simulink model "fivephase_inverter_without_speed_control_v66"  (R2019b)
settings: Solver=FixedStepAuto  StartTime=0.0  StopTime=0.2  FixedStep=t_s  MaxStep=1e-4  RelTol=1e-3
values from neighbouring files (symbols this model uses):
  pulse = zeros(5,7,10)    [run_simulink_model.m]
  T_load_time = 0    [run_simulink_model.m]
  t_s = 1e-6    (= 1e-06)    [run_simulink_model.m]
  w_init = 70*pi    (= 219.911485751)    [run_simulink_model.m]
  w_rev_time = 3    [run_simulink_model.m]
  w_set = 70*pi    (= 219.911485751)    [run_simulink_model.m]
libraries: powerlib x49, simulink x6, powerlib_meascontrol x5, simulink_extras x1
settings Model: Creator=user  LastModifiedBy=user
settings SolverCC: AlgebraicLoopSolver=LineSearch
settings DataIOCC: ReturnWorkspaceOutputs=off
settings DebuggingCC: ArithmeticOperatorsInVariantConditions=warning
settings SFSimCC: SimUseLocalCustomCode=off  CustomCodeUndefinedFunction=UseInterfaceOnly
settings RTWCC: RTWUseLocalCustomCode=off

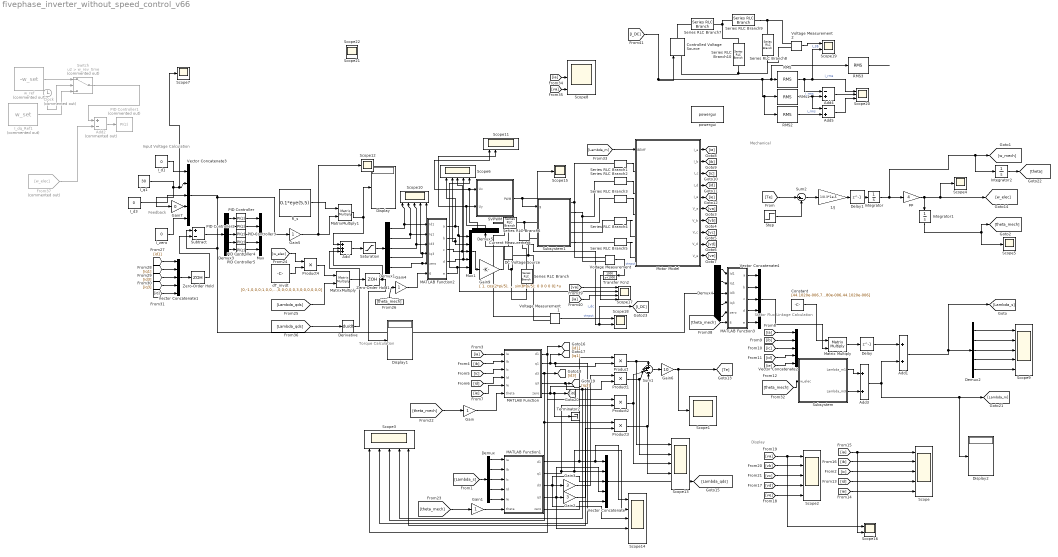
== system fivephase_inverter_without_speed_control_v66 ==
  note: Input Voltage Calculation
  note: Feedback
  note: Torque Calculation
  note: Stator Flux Linkage Calculation
  note: Mechanical
  note: Display
  1/J : Gain  Gain=1/0.3*1e-5
  Add : Sum  Inputs=+++
  Add1 : Sum
  Add2 : Sum  Commented=on  Inputs=+-
  Add3 : Sum
  Add4 : Sum  Inputs=-+
  Add5 : Sum  Inputs=-+
  Clock : Clock  Commented=on
  Constant : Constant  Value=[44.1020e-006,7.6280e-006,-24.9980e-006,-24.9980e-006,7.6280e-006;7.6280e-006,44.1020e-006,7.6280e-006,-24.9980e-006,-24.9980e-006;-24.9980e-006,7.6280e-006, 44.1020e-006,7.6280e-006,-24.9980e-006;-24.9980e-006,-24.9980e-006,7.6280e-006,44.1020e-006,7.6280e-006;7.6280e-006 ,-24.9980e-006,-24.9980e-006,7.6280e-006,44.1020e-006]  SampleTime=-1
  Controlled Voltage Source : powerlib/Electrical Sources/Controlled Voltage Source  Initialize=on  Source_Type=AC  Amplitude=0  Phase=0  Frequency=0  Measurements=None
      settings: SourceProductName=Simscape Electrical
  Current Measurement : powerlib/Measurements/Current Measurement  PhasorSimulation=off  OutputType=Complex  PSBequivalent=0
      settings: SourceProductName=Simscape Electrical
  DC Voltage Source : powerlib/Electrical Sources/DC Voltage Source  Amplitude=80  Measurements=None
      settings: SourceProductName=Simscape Electrical
  Delay : Delay  DelayLength=1  InitialCondition=1
  Delay1 : Delay  DelayLength=1  InitialCondition=35/2*pi
  Demux{,1..4} (5 alike) : Demux  Outputs=5
  Demux5 : Demux  Outputs=3
  Derivative : Derivative  CoefficientInTFapproximation=1e-5
  Display : Display
  Display1 : Display
  Display2 : Display
  From37 : From  Commented=on  GotoTag=w_elec
  Gain{,1,4..5} (4 alike) : Gain
  Gain2 : Gain  Gain=3
  Gain3 : Gain  Gain=3
  Gain6 : Gain  Gain=10
  Gain7 : Gain  Gain=0
  Gain9 : Gain  Gain=[ 1, cos(2*pi/5), cos(4*pi/5), cos(6*pi/5), cos(8*pi/5); 0, sin(2*pi/5),sin(4*pi/5), sin(6*pi/5), sin(8*pi/5); 0 0 0 0 0]  Multiplication=Matrix(K*u) (u vector)  SaturateOnIntegerOverflow=on  OutDataTypeStr=Inherit: Same as input  ParamDataTypeStr=Inherit: Same as input
  I_d1 : Constant  Value=0
  I_d3 : Constant  Value=0
  I_dq_Ref1 : Constant  Commented=on  Value=w_set
  I_q1 : Constant  Value=30
  I_zero : Constant  Value=0
  Integrator : Integrator  InitialCondition=w_init/4
  Integrator1 : Integrator
  Integrator2 : Integrator
  MATLAB Function : MATLAB Function  TreatAsAtomicUnit=on
  MATLAB Function1 : MATLAB Function  TreatAsAtomicUnit=on
  MATLAB Function2 : MATLAB Function  TreatAsAtomicUnit=on
  MATLAB Function3 : MATLAB Function  TreatAsAtomicUnit=on
  Matrix Multiply : Product  Multiplication=Matrix(*)
  MatrixMultiply : Product  Multiplication=Matrix(*)
  MatrixMultiply1 : Product  Multiplication=Matrix(*)
  Motor Model : Subsystem
  Mux : Mux  Inputs=5
  Mux1 : Mux  Inputs=5
  PID Controller{,2..5} (5 alike) : simulink/Continuous/PID Controller  Controller=PI  Form=Parallel  TimeDomain=Discrete-time  SampleTime=t_s  IntegratorMethod=Forward Euler  FilterMethod=Forward Euler  ControllerParametersSource=internal  P=5  I=5  D=0  UseFilter=on  N=100  TunerSelectOption=Transfer Function Based (PID Tuner App)  InitialConditionSource=internal  InitialConditionForIntegrator=0  InitialConditionForFilter=0  DifferentiatorICPrevScaledInput=0  ExternalReset=none  TrackingMode=off  Kt=1  LimitOutput=off  UpperSaturationLimit=75  LowerSaturationLimit=-75  LinearizeAsGain=on  AntiWindupMode=clamping  Kb=1  POutMin=[]  POutMax=[]  IOutMin=[]  IOutMax=[]  DOutMin=[]  DOutMax=[]  NOutMin=[]  NOutMax=[]  SumOutMin=[]  SumOutMax=[]  SaturationOutMin=[]  SaturationOutMax=[]  PParamMin=[]  PParamMax=[]  IParamMin=[]  IParamMax=[]  DParamMin=[]  DParamMax=[]  NParamMin=[]  NParamMax=[]  KbParamMin=[]  KbParamMax=[]  KtParamMin=[]  KtParamMax=[]  KbOutMin=[]  KbOutMax=[]  KtOutMin=[]  KtOutMax=[]  IntegratorOutMin=[]  IntegratorOutMax=[]  FilterOutMin=[]  FilterOutMax=[]  SumI1OutMin=[]  SumI1OutMax=[]  SumI2OutMin=[]  SumI2OutMax=[]  SumI3OutMin=[]  SumI3OutMax=[]  SumI4OutMin=[]  SumI4OutMax=[]  SumDOutMin=[]  SumDOutMax=[]  DifferentiatorOutMin=[]  DifferentiatorOutMax=[]  FilterDiffOutCoefMin=[]  FilterDiffOutCoefMax=[]  ReciprocalOutMin=[]  ReciprocalOutMax=[]  SumDenOutMin=[]  SumDenOutMax=[]  SumNumOutMin=[]  SumNumOutMax=[]  DivideOutMin=[]  DivideOutMax=[]  IntegratorContinuousStateAttributes=''  IntegratorStateMustResolveToSignalObject=off  IntegratorRTWStateStorageClass=Auto  FilterContinuousStateAttributes=''  FilterStateMustResolveToSignalObject=off  FilterRTWStateStorageClass=Auto  ParallelPVariant=InternalParameters  IdealPVariant=Disabled  IVariant=InternalParameters  DVariant=Disabled  IntegratorVariant=Discrete  SatVariant=Disabled  AWVariant=Passthrough  PCopyVariant=Disabled  TRVariant=Disabled  FdbkBlocksVariant=Forward  IdealPFdbkVariant=Disabled  SatFdbkVariant=Disabled  DerivativeFilterVariant=Disabled  NVariant=Disabled  NCopyVariant=Disabled_SignalSpec  FilterICVariant=Disabled  IntegratorICVariant=InternalICs  ExternalResetVariant=Disabled  TRSumVariant=Passthrough  SumFdbkVariant=Disabled  SumVariant=Sum_PI
  PID Controller1 : simulink/Continuous/PID Controller  Commented=on  Controller=PI  Form=Parallel  TimeDomain=Discrete-time  SampleTime=t_s  IntegratorMethod=Forward Euler  FilterMethod=Forward Euler  ControllerParametersSource=internal  P=2  I=30  D=0  UseFilter=on  N=100  TunerSelectOption=Transfer Function Based (PID Tuner App)  InitialConditionSource=internal  InitialConditionForIntegrator=0  InitialConditionForFilter=0  DifferentiatorICPrevScaledInput=0  ExternalReset=none  TrackingMode=off  Kt=1  LimitOutput=on  UpperSaturationLimit=80  LowerSaturationLimit=-80  LinearizeAsGain=on  AntiWindupMode=clamping  Kb=1  POutMin=[]  POutMax=[]  IOutMin=[]  IOutMax=[]  DOutMin=[]  DOutMax=[]  NOutMin=[]  NOutMax=[]  SumOutMin=[]  SumOutMax=[]  SaturationOutMin=[]  SaturationOutMax=[]  PParamMin=[]  PParamMax=[]  IParamMin=[]  IParamMax=[]  DParamMin=[]  DParamMax=[]  NParamMin=[]  NParamMax=[]  KbParamMin=[]  KbParamMax=[]  KtParamMin=[]  KtParamMax=[]  KbOutMin=[]  KbOutMax=[]  KtOutMin=[]  KtOutMax=[]  IntegratorOutMin=[]  IntegratorOutMax=[]  FilterOutMin=[]  FilterOutMax=[]  SumI1OutMin=[]  SumI1OutMax=[]  SumI2OutMin=[]  SumI2OutMax=[]  SumI3OutMin=[]  SumI3OutMax=[]  SumI4OutMin=[]  SumI4OutMax=[]  SumDOutMin=[]  SumDOutMax=[]  DifferentiatorOutMin=[]  DifferentiatorOutMax=[]  FilterDiffOutCoefMin=[]  FilterDiffOutCoefMax=[]  ReciprocalOutMin=[]  ReciprocalOutMax=[]  SumDenOutMin=[]  SumDenOutMax=[]  SumNumOutMin=[]  SumNumOutMax=[]  DivideOutMin=[]  DivideOutMax=[]  IntegratorContinuousStateAttributes=''  IntegratorStateMustResolveToSignalObject=off  IntegratorRTWStateStorageClass=Auto  FilterContinuousStateAttributes=''  FilterStateMustResolveToSignalObject=off  FilterRTWStateStorageClass=Auto  ParallelPVariant=InternalParameters  IdealPVariant=Disabled  IVariant=InternalParameters  DVariant=Disabled  IntegratorVariant=Discrete  SatVariant=Enabled  AWVariant=DiscClampingParallel  PCopyVariant=Disabled  TRVariant=Disabled  FdbkBlocksVariant=Forward  IdealPFdbkVariant=Disabled  SatFdbkVariant=Disabled  DerivativeFilterVariant=Disabled  NVariant=Disabled  NCopyVariant=Disabled_SignalSpec  FilterICVariant=Disabled  IntegratorICVariant=InternalICs  ExternalResetVariant=Disabled  TRSumVariant=Passthrough  SumFdbkVariant=Disabled  SumVariant=Sum_PI
  Product{,1..4} (5 alike) : Product
  RMS : powerlib_meascontrol/Measurements/RMS  TrueRMS=off  Freq=350  RMSInit=0  Ts=0
      settings: SourceProductName=Simscape Electrical
  RMS1 : powerlib_meascontrol/Measurements/RMS  TrueRMS=off  Freq=700  RMSInit=0  Ts=0
      settings: SourceProductName=Simscape Electrical
  RMS2 : powerlib_meascontrol/Measurements/RMS  TrueRMS=off  Freq=15000  RMSInit=0  Ts=0
      settings: SourceProductName=Simscape Electrical
  RMS3 : powerlib_meascontrol/Measurements/RMS  TrueRMS=off  Freq=7  RMSInit=0  Ts=0
      settings: SourceProductName=Simscape Electrical
  R_s : Constant  Value=0.1*eye(5,5)
  SVPWM : Subsystem  mask{Fc=15000, Vdc=80, Ts=t_s}
      mask prompts: Fc "PWM frequency"; Vdc "DC bus voltage"; Ts "Sampling time"
  Saturation : Saturate  UpperLimit=50  LowerLimit=-50
  Scope{,2..3,6,9..11,13..14} (9 alike) : Scope  NumInputPorts=5
  Scope{1,4..5,7,12,15,21..22} (8 alike) : Scope
  Scope16 : Scope  NumInputPorts=2
  Scope17 : Scope  NumInputPorts=4
  Scope18 : Scope  NumInputPorts=2
  Scope19 : Scope  NumInputPorts=2
  Scope20 : Scope  NumInputPorts=3
  Scope8 : Scope  NumInputPorts=3
  Series RLC Branch : powerlib/Elements/Series RLC Branch  LConnTagsString=__new0  RConnTagsString=__new0  BranchType=RC  Resistance=1e-12  Inductance=1e-3  SetiL0=off  InitialCurrent=0  Capacitance=100e-6  Setx0=off  InitialVoltage=0  Measurements=None
      settings: SourceProductName=Simscape Electrical
  Series RLC Branch{1..5} (5 alike) : powerlib/Elements/Series RLC Branch  LConnTagsString=__new0  RConnTagsString=__new0  BranchType=R  Resistance=1e-2  Inductance=1e-3  SetiL0=off  InitialCurrent=0  Capacitance=1e-6  Setx0=off  InitialVoltage=0  Measurements=None
      settings: SourceProductName=Simscape Electrical
  Series RLC Branch10 : powerlib/Elements/Series RLC Branch  LConnTagsString=__new0  RConnTagsString=__new0  BranchType=C  Resistance=50  Inductance=125.6e-3  SetiL0=off  InitialCurrent=0  Capacitance=5.025e-6  Setx0=off  InitialVoltage=0  Measurements=None
      settings: SourceProductName=Simscape Electrical
  Series RLC Branch6 : powerlib/Elements/Series RLC Branch  LConnTagsString=__new0  RConnTagsString=__new0  BranchType=L  Resistance=1e-12  Inductance=1e-3  SetiL0=off  InitialCurrent=0  Capacitance=100e-6  Setx0=off  InitialVoltage=0  Measurements=None
      settings: SourceProductName=Simscape Electrical
  Series RLC Branch7 : powerlib/Elements/Series RLC Branch  LConnTagsString=__new0  RConnTagsString=__new0  BranchType=R  Resistance=50  Inductance=1e-3  SetiL0=off  InitialCurrent=0  Capacitance=1e-6  Setx0=off  InitialVoltage=0  Measurements=None
      settings: SourceProductName=Simscape Electrical
  Series RLC Branch8 : powerlib/Elements/Series RLC Branch  LConnTagsString=__new0  RConnTagsString=__new0  BranchType=R  Resistance=50  Inductance=1e-3  SetiL0=off  InitialCurrent=0  Capacitance=1e-6  Setx0=off  InitialVoltage=0  Measurements=None
      settings: SourceProductName=Simscape Electrical
  Series RLC Branch9 : powerlib/Elements/Series RLC Branch  LConnTagsString=__new0  RConnTagsString=__new0  BranchType=L  Resistance=50  Inductance=12.56e-3  SetiL0=off  InitialCurrent=0  Capacitance=1e-6  Setx0=off  InitialVoltage=0  Measurements=None
      settings: SourceProductName=Simscape Electrical
  Step : Step  Time=T_load_time  After=26.07  SampleTime=0
  Subsystem : Subsystem
  Subsystem1 : Subsystem
  Subtract : Sum  Inputs=+-
  Sum1 : Sum  Inputs=++--
  Sum2 : Sum  Inputs=|+-
  Switch : Switch  Commented=on  Criteria=u2 > Threshold  Threshold=w_rev_time
  Terminator2 : Terminator
  Transfer Fcn2 : TransferFcn  Numerator=[1000]  Denominator=[1 1000]
  Vector Concatenate{,1..4} (5 alike) : Concatenate  NumInputs=5
  Voltage Measurement : powerlib/Measurements/Voltage Measurement  PhasorSimulation=off  OutputType=Complex  PSBequivalent=0
      settings: SourceProductName=Simscape Electrical
  Voltage Measurement1 : powerlib/Measurements/Voltage Measurement  PhasorSimulation=off  OutputType=Complex  PSBequivalent=0
      settings: SourceProductName=Simscape Electrical
  Voltage Measurement2 : powerlib/Measurements/Voltage Measurement  PhasorSimulation=off  OutputType=Complex  PSBequivalent=0
      settings: SourceProductName=Simscape Electrical
  Zero-Order Hold : ZeroOrderHold  SampleTime=-1
  Zero-Order Hold1 : ZeroOrderHold  SampleTime=-1
  dT_invdt : Constant  Value=[0,-1,0,0,0;1,0,0,0,0;0,0,-3,0,0;0,0,0,3,0;0,0,0,0,0]
  powergui : powerlib/powergui  Priority=1  SimulationMode=Discrete  SampleTime=t_s  frequency=60  Iterations=50  frequencyindice=0  Pbase=100e6  ErrMax=1e-4  UnitsV=kV  UnitsW=MW  buscounter=0  FunctionMessages=off  echomessages=off  EnableUseOfTLC=off  CurrentSourceSwitches=off  DisableSnubberDevices=off  DisableRonSwitches=off  DisableVfSwitches=off  DisplayEquations=off  AutomaticDiscreteSolvers=off  SolverType=Tustin/Backward Euler (TBE)  Interpol=off  ExternalGateDelay=off  methode=off  Ts=100  x0status=blocks  SPID=on  SwTol=0  HookPort=off  NonlinearTolerance=1e-4  nMaxIteration=100  ContinueOnMaxIteration=off  RestoreLinks=warning  ResistiveCurrentMeasurement=off  Frange=[0:2:500]  Ylog=off  Xlog=on  ShowGrid=off  save=off  variable=ZData  structure=logsout  ZoomFFT=off  StartTime=0.04  cycles=20  DisplayStyle=1  fundamental=15000  FreqAxis=on  MaxFrequency=150000  frequencyindicesteady=1  RmsSteady=1  display=off
      settings: SourceProductName=Simscape Electrical
  pp : Gain  Gain=4
  w_ref : Constant  Commented=on  Value=-w_set
  wires:
  [ia] -> MATLAB Function/1(Ia)
  [ib] -> MATLAB Function/2(Ib)
  [ic] -> MATLAB Function/3(Ic)
  [id] -> MATLAB Function/4(Id)
  [ie] -> MATLAB Function/5(Ie)
  MATLAB Function/1(d1) -> Product2/1, Scope3/1, [id1]
  MATLAB Function/3(d3) -> Product3/1, Scope3/3, [id3]
  MATLAB Function/5(zero) -> [i0], Terminator2/1, Scope3/5
  MATLAB Function/2(q1) -> [iq1], Product/2, Scope3/2
  MATLAB Function1/1(d1) -> Scope14/1, Vector Concatenate/1, Product/1
  Gain3/1 -> Product1/1
  MATLAB Function/4(q3) -> Product1/2, Scope3/4, [iq3]
  Product/1 -> Scope13/1, Sum1/1
  Product1/1 -> Scope13/2, Sum1/2
  Sum1/1 -> Gain6/1
  [ib] -> Scope/2
  [ia] -> Scope/1, Scope16/2
  [id] -> Scope/4
  [ic] -> Scope/3
  [ie] -> Scope/5
  [ve] -> Scope2/5
  [vd] -> Scope2/4
  [vc] -> Scope2/3
  [vb] -> Scope2/2
  [va] -> Scope16/1, Scope2/1
  [Te] -> Sum2/1
  Step/1 -> Sum2/2
  Sum2/1 -> 1/J/1
  Integrator/1 -> Integrator2/1, [w_mech], pp/1
  Gain/1 -> MATLAB Function/6(theta)
  [theta_mech] -> Gain/1
  [ia] -> Vector Concatenate2/1
  [ib] -> Vector Concatenate2/2
  [ic] -> Vector Concatenate2/3
  [id] -> Vector Concatenate2/4
  [ie] -> Vector Concatenate2/5
  Constant/1 -> Matrix Multiply/1
  Add1/1 -> [Lambda_s], Demux2/1
  [Lambda_s] -> Demux/1
  Demux/1 -> MATLAB Function1/1(Ia)
  Demux/2 -> MATLAB Function1/2(Ib)
  Demux/3 -> MATLAB Function1/3(Ic)
  Demux/4 -> MATLAB Function1/4(Id)
  Demux/5 -> MATLAB Function1/5(Ie)
  [theta_mech] -> Gain1/1
  Gain1/1 -> MATLAB Function1/6(theta)
  MATLAB Function1/3(d3) -> Scope14/3, Vector Concatenate/3, Gain3/1
  MATLAB Function1/4(q3) -> Scope14/4, Vector Concatenate/4, Gain2/1
  Gain2/1 -> Product3/2
  MATLAB Function1/2(q1) -> Scope14/2, Vector Concatenate/2, Product2/2
  Product2/1 -> Sum1/3, Scope13/3
  Product3/1 -> Scope13/4, Sum1/4
  Motor Model/6(V_a) -> [va]
  Motor Model/7(V_b) -> [vb]
  Motor Model/8(V_c) -> [vc]
  Motor Model/9(V_d) -> [vd]
  Motor Model/10(V_e) -> [ve]
  Motor Model/1(I_a) -> [ia]
  Motor Model/2(I_b) -> [ib]
  Motor Model/3(I_c) -> [ic]
  Motor Model/4(I_d) -> [id]
  Motor Model/5(I_e) -> [ie]
  [w_elec] -> Product4/1
  dT_invdt/1 -> Product4/2
  MATLAB Function1/5(zero) -> Vector Concatenate/5
  Vector Concatenate/1 -> [Lambda_qds]
  Product4/1 -> MatrixMultiply/1
  [Lambda_qds] -> MatrixMultiply/2
  R_s/1 -> MatrixMultiply1/1
  MatrixMultiply1/1 -> Display/1, Add/1
  Add/1 -> Saturation/1
  Demux1/5 -> Scope10/5, MATLAB Function2/5(zero)
  [theta_mech] -> Gain4/1
  Gain4/1 -> MATLAB Function2/6(theta)
  [id1] -> Vector Concatenate1/1
  [iq1] -> Vector Concatenate1/2
  [id3] -> Vector Concatenate1/3
  [iq3] -> Vector Concatenate1/4
  [i0] -> Vector Concatenate1/5
  Gain5/1 -> Scope12/1, MatrixMultiply1/2
  [theta_mech] -> Subsystem/1("w_elec ")
  Vector Concatenate1/1 -> Zero-Order Hold/1
  Zero-Order Hold1/1 -> Display1/1, Add/2
  MatrixMultiply/1 -> Zero-Order Hold1/1
  Matrix Multiply/1 -> Delay/1
  1/J/1 -> Delay1/1
  Delay1/1 -> Integrator/1
  Subsystem/1(Lambda_m1) -> Add3/1
  Subsystem/2(Lambda_m3) -> Add3/2
  [Lambda_m] -> Motor Model/1(BEMF)
  pp/1 -> Scope4/1, [w_elec], Integrator1/1
  [ia] -> Scope8/2
  [va] -> Scope8/3
  [Lambda_qds] -> Derivative/1
  Derivative/1 -> Add/3
  Delay/1 -> Add1/1
  Gain6/1 -> [Te], Scope1/1
  Integrator2/1 -> [theta]
  Add3/1 -> Display2/1, [Lambda_m], Add1/2
  Demux2/1 -> Scope9/1
  Demux2/2 -> Scope9/2
  Demux2/3 -> Scope9/3
  Demux2/4 -> Scope9/4
  Demux2/5 -> Scope9/5
  Demux1/1 -> Scope10/1, MATLAB Function2/1(Id1)
  Demux1/2 -> Scope10/2, MATLAB Function2/2(Iq1)
  Demux1/3 -> Scope10/3, MATLAB Function2/3(Id3)
  Demux1/4 -> Scope10/4, MATLAB Function2/4(Iq3)
  Vector Concatenate3/1 -> Gain5/1, Subtract/1, Demux4/1
  From37/1 -> Add2/2
  I_dq_Ref1/1 -> Switch/3
  Clock/1 -> Switch/2
  Add2/1 -> PID Controller1/1
  I_q1/1 -> Gain7/1, Scope7/1, Vector Concatenate3/2
  I_d1/1 -> Vector Concatenate3/1
  I_d3/1 -> Vector Concatenate3/3
  I_zero/1 -> Vector Concatenate3/5
  w_ref/1 -> Switch/1
  Switch/1 -> Add2/1
  Demux3/1 -> PID Controller/1
  Demux3/2 -> PID Controller2/1
  Demux3/3 -> PID Controller3/1
  Demux3/4 -> PID Controller4/1
  Demux3/5 -> PID Controller5/1
  PID Controller/1 -> Mux/1
  PID Controller2/1 -> Mux/2
  PID Controller3/1 -> Mux/3
  PID Controller4/1 -> Mux/4
  PID Controller5/1 -> Mux/5
  Gain7/1 -> Vector Concatenate3/4
  [theta_mech] -> MATLAB Function3/6(theta)
  Demux4/1 -> MATLAB Function3/1(Id1)
  Demux4/2 -> MATLAB Function3/2(Iq1)
  Demux4/3 -> MATLAB Function3/3(Id3)
  Demux4/4 -> MATLAB Function3/4(Iq3)
  Demux4/5 -> MATLAB Function3/5(zero)
  MATLAB Function3/1(a) -> Vector Concatenate4/1
  MATLAB Function3/2(b) -> Vector Concatenate4/2
  MATLAB Function3/3(c) -> Vector Concatenate4/3
  MATLAB Function3/4(d) -> Vector Concatenate4/4
  MATLAB Function3/5(e) -> Vector Concatenate4/5
  Zero-Order Hold/1 -> Subtract/2
  Subtract/1 -> Demux3/1
  SVPWM/1(PWM) -> Scope15/1, Subsystem1/1(g)
  Mux1/1 -> Gain9/1
  Gain9/1 -> Demux5/1
  MATLAB Function2/1(a) -> Scope6/1, Scope17/2, Mux1/1
  MATLAB Function2/2(b) -> Scope6/2, Mux1/2
  MATLAB Function2/4(d) -> Scope6/4, Mux1/4
  MATLAB Function2/3(c) -> Scope6/3, Mux1/3
  MATLAB Function2/5(e) -> Mux1/5, Scope6/5
  Demux5/1 -> SVPWM/1(Ux), Scope11/1
  Demux5/2 -> SVPWM/2(Uy), Scope11/2
  [va] -> Scope17/1
  [ia] -> Scope17/3
  Voltage Measurement/1 -> Transfer Fcn2/1  "vinput"
  Transfer Fcn2/1 -> Scope17/4
  Integrator1/1 -> [theta_mech], Scope5/1
  Vector Concatenate4/1 -> Matrix Multiply/2
  Saturation/1 -> Demux1/1
  Voltage Measurement1/1 -> Scope18/1  "vinput"
  Current Measurement/1 -> [I_DC], Scope18/2  "i_dc"
  [I_DC] -> Controlled Voltage Source/1, RMS2/1, RMS1/1, RMS3/1, RMS/1
  Voltage Measurement2/1 -> Scope19/1  "I_35"
  RMS/1 -> Add4/1, Scope20/1, Scope19/2  "i_rms"
  RMS1/1 -> Add5/1, Add4/2  "i_rms"
  RMS2/1 -> Add5/2  "i_rms"
  Add5/1 -> Scope20/3
  Add4/1 -> Scope20/2
  RMS3/1 -> ?
  connections:
  Series RLC Branch1/RConn1 -- Motor Model/LConn1
  Series RLC Branch2/RConn1 -- Motor Model/LConn2
  Series RLC Branch3/RConn1 -- Motor Model/LConn3
  Series RLC Branch4/RConn1 -- Motor Model/LConn4
  Series RLC Branch5/RConn1 -- Motor Model/LConn5
  Series RLC Branch1/LConn1 -- Voltage Measurement/LConn1 -- Subsystem1/RConn1
  Subsystem1/LConn2 -- Series RLC Branch/RConn1 -- DC Voltage Source/LConn1 -- Voltage Measurement1/LConn2
  Series RLC Branch3/LConn1 -- Subsystem1/RConn3
  Subsystem1/RConn2 -- Voltage Measurement/LConn2 -- Series RLC Branch2/LConn1
  Series RLC Branch4/LConn1 -- Subsystem1/RConn4
  Series RLC Branch6/LConn1 -- DC Voltage Source/RConn1 -- Voltage Measurement1/LConn1
  Subsystem1/LConn1 -- Current Measurement/LConn1 -- Series RLC Branch6/RConn1
  Series RLC Branch/LConn1 -- Current Measurement/RConn1
  Series RLC Branch7/LConn1 -- Controlled Voltage Source/RConn1
  Series RLC Branch9/LConn1 -- Series RLC Branch7/RConn1 -- Series RLC Branch10/LConn1
  Series RLC Branch9/RConn1 -- Voltage Measurement2/LConn1 -- Series RLC Branch8/LConn1
  Series RLC Branch10/RConn1 -- Voltage Measurement2/LConn2 -- Series RLC Branch8/RConn1 -- Controlled Voltage Source/LConn1
  Subsystem1/RConn5 -- Series RLC Branch5/LConn1

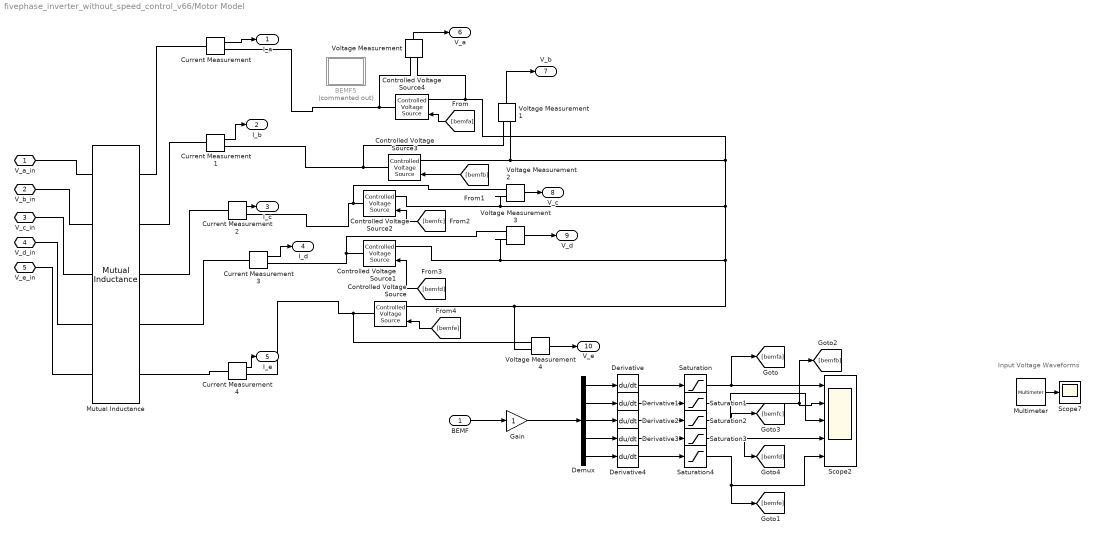
== system fivephase_inverter_without_speed_control_v66/Motor Model ==
  note: Input Voltage Waveforms
  BEMF : Inport
  BEMF5 : Subsystem  Commented=on  mask{freq=35, fund=20, third=0, fifth=0, phase=0}
      mask prompts: freq "Frequency"; fund "Fundamental Magnitude"; third "Third Harmonic"; fifth "Fifth Harmonic"
  Controlled Voltage Source{,1..4} (5 alike) : powerlib/Electrical Sources/Controlled Voltage Source  Initialize=on  Source_Type=AC  Amplitude=0  Phase=0  Frequency=0  Measurements=Voltage
      settings: SourceProductName=Simscape Electrical
  Current Measurement{,1..4} (5 alike) : powerlib/Measurements/Current Measurement  PhasorSimulation=off  OutputType=Complex  PSBequivalent=0
      settings: SourceProductName=Simscape Electrical
  Demux : Demux  Outputs=5
  Derivative{,1..4} (5 alike) : Derivative
  Gain : Gain
  Multimeter : powerlib/Measurements/Multimeter  PhasorSimulation=off  OutputType=Complex  sel=[8 10 7 9 6]  L=15  Gain=[1 1 1 1 1]  yselected={'Usrc: Motor Model/Controlled Voltage Source2','Usrc: Motor Model/Controlled Voltage Source4','Usrc: Motor Model/Controlled Voltage Source1','Usrc: Motor Model/Controlled Voltage Source3','Usrc: Motor Model/Controlled Voltage Source'};  PSBOutputType=1  PSBequivalent=0  AxesSetting=[0,0.1,-100,100]  Display=0  SavedBlockNames=-11
      settings: SourceProductName=Simscape Electrical
  Mutual Inductance : powerlib/Elements/Mutual Inductance  LConnTagsString=a|b|c|L4|L5  RConnTagsString=A|B|C|R4|R5  TypeOfMutual=Generalized mutual inductance  NumberOfWindings=5  SelfImpedance1=[1.1 1.1e-03]  SelfImpedance2=[ 1.1 1.1e-03]  ThreeWindings=on  SelfImpedance3=[ 1.1 1.1e-03]  MutualImpedance=[1.0 1.0e-03]  InductanceMatrix=L_an  ResistanceMatrix=[1e-5,0,0,0,0 ; 0,1e-5,0,0,0; 0,0,1e-5,0,0; 0,0,0,1e-5,0; 0,0,0,0,1e-5]*1e4  Measurements=Winding voltages and currents
      settings: AttributesFormatString=\n  SourceProductName=Simscape Electrical  SourceProductBaseCode=PS
  Saturation{,1..4} (5 alike) : Saturate  UpperLimit=50  LowerLimit=-50
  Scope2 : Scope  NumInputPorts=5
  Scope7 : Scope
  Voltage Measurement{,1..4} (5 alike) : powerlib/Measurements/Voltage Measurement  PhasorSimulation=off  OutputType=Complex  PSBequivalent=0
      settings: SourceProductName=Simscape Electrical
  V_a_in : PMIOPort  Side=Left
  V_b_in : PMIOPort  Port=2  Side=Left
  V_c_in : PMIOPort  Port=3  Side=Left
  V_d_in : PMIOPort  Port=4  Side=Left
  V_e_in : PMIOPort  Port=5  Side=Left
  I_a : Outport
  I_b : Outport  Port=2
  I_c : Outport  Port=3
  I_d : Outport  Port=4
  I_e : Outport  Port=5
  V_a : Outport  Port=6
  V_b : Outport  Port=7
  V_c : Outport  Port=8
  V_d : Outport  Port=9
  V_e : Outport  Port=10
  wires:
  Current Measurement/1 -> I_a/1
  Current Measurement3/1 -> I_d/1
  Current Measurement1/1 -> I_b/1
  Current Measurement2/1 -> I_c/1
  Voltage Measurement2/1 -> V_c/1
  Voltage Measurement/1 -> V_a/1
  Current Measurement4/1 -> I_e/1
  Voltage Measurement1/1 -> V_b/1
  Voltage Measurement4/1 -> V_e/1
  Voltage Measurement3/1 -> V_d/1
  Demux/1 -> Derivative/1
  Demux/2 -> Derivative1/1
  Demux/3 -> Derivative2/1
  Demux/4 -> Derivative3/1
  Demux/5 -> Derivative4/1
  Derivative/1 -> Saturation/1
  [bemfa] -> Controlled Voltage Source4/1
  [bemfb] -> Controlled Voltage Source3/1
  [bemfc] -> Controlled Voltage Source2/1
  [bemfd] -> Controlled Voltage Source1/1
  [bemfe] -> Controlled Voltage Source/1
  Derivative4/1 -> Saturation4/1
  Derivative1/1 -> Saturation1/1
  Derivative2/1 -> Saturation2/1
  Derivative3/1 -> Saturation3/1
  BEMF/1 -> Gain/1
  Gain/1 -> Demux/1
  Saturation/1 -> Scope2/1, [bemfa]
  Saturation2/1 -> Scope2/3, [bemfc]
  Saturation3/1 -> Scope2/4, [bemfd]
  Saturation4/1 -> Scope2/5, [bemfe]
  Saturation1/1 -> Scope2/2, [bemfb]
  Multimeter/1 -> Scope7/1
  connections:
  Controlled Voltage Source/LConn1 -- Voltage Measurement4/LConn2 -- Voltage Measurement/LConn2 -- Controlled Voltage Source4/LConn1 -- Voltage Measurement1/LConn2 -- Controlled Voltage Source3/LConn1 -- Voltage Measurement2/LConn2 -- Controlled Voltage Source2/LConn1 -- Voltage Measurement3/LConn2 -- Controlled Voltage Source1/LConn1
  Controlled Voltage Source2/RConn1 -- Current Measurement2/RConn1 -- Voltage Measurement2/LConn1
  Controlled Voltage Source/RConn1 -- Voltage Measurement4/LConn1 -- Current Measurement4/RConn1
  Controlled Voltage Source4/RConn1 -- Voltage Measurement/LConn1 -- Current Measurement/RConn1
  Mutual Inductance/RConn1 -- Current Measurement/LConn1
  Controlled Voltage Source1/RConn1 -- Current Measurement3/RConn1 -- Voltage Measurement3/LConn1
  Current Measurement1/LConn1 -- Mutual Inductance/RConn2
  Current Measurement3/LConn1 -- Mutual Inductance/RConn4
  Current Measurement1/RConn1 -- Voltage Measurement1/LConn1 -- Controlled Voltage Source3/RConn1
  Current Measurement2/LConn1 -- Mutual Inductance/RConn3
  Current Measurement4/LConn1 -- Mutual Inductance/RConn5
  V_e_in/RConn1 -- Mutual Inductance/LConn5
  V_d_in/RConn1 -- Mutual Inductance/LConn4
  V_c_in/RConn1 -- Mutual Inductance/LConn3
  V_b_in/RConn1 -- Mutual Inductance/LConn2
  V_a_in/RConn1 -- Mutual Inductance/LConn1

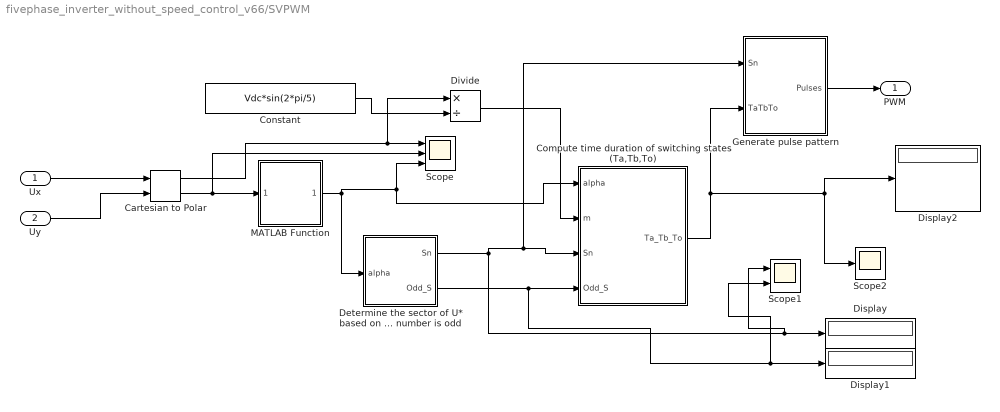
== system fivephase_inverter_without_speed_control_v66/SVPWM ==
  Ux : Inport
  Uy : Inport  Port=2
  Cartesian to Polar : simulink_extras/Transformations/Cartesian to Polar
      settings: SourceProductName=Simulink
  "Compute time duration of switching states (Ta,Tb,To) " : Subsystem  AncestorBlock=|
      | spsSVPWMGenerator2LevelModel/Continuous/SV Modulator
      | Pattern #1/Compute time duration of
      | switching states (Ta,Tb,To)
  Constant : Constant  Value=Vdc*sin(2*pi/5)
  "Determine the sector of U* based on alpha (rad). Also, determine if the sector number is odd" : Subsystem  AncestorBlock=|
      | spsSVPWMGenerator2LevelModel/Continuous/SV Modulator
      | Pattern #1/Determine the sector of U*
      | based on alpha (rad). Also, determine
      | if the sector number is odd
  Display : Display
  Display1 : Display
  Display2 : Display
  Divide : Product  Inputs=*/
  Generate pulse pattern : Subsystem  AncestorBlock=|
      | spsSVPWMGenerator2LevelModel/Discrete/SV Modulator
      | Pattern #1/Generate 
      | pulse pattern
      mask init:
      | %Switching pattern:
      | pat1=[0 1 1 1 1 1 0;0 0 1 1 1 0 0;0 0 0 1 0 0 0];
      | pat1(:,:,2)=[0 0 1 1 1 0 0;0 1 1 1 1 1 0;0 0 0 1 0 0 0];
      | pat1(:,:,3)=[0 0 0 1 0 0 0;0 1 1 1 1 1 0;0 0 1 1 1 0 0];
      | pat1(:,:,4)=[0 0 0 1 0 0 0;0 0 1 1 1 0 0;0 1 1 1 1 1 0];
      | pat1(:,:,5)=[0 0 1 1 1 0 0;0 0 0 1 0 0 0;0 1 1 1 1 1 0];
      | pat1(:,:,6)=[0 1 1 1 1 1 0;0 0 0 1 0 0 0;0 0 1 1 1 0 0];
  MATLAB Function : MATLAB Function  TreatAsAtomicUnit=on
  Scope : Scope  NumInputPorts=3
  Scope1 : Scope  NumInputPorts=2
  Scope2 : Scope
  PWM : Outport
  wires:
  Generate pulse pattern/1(Pulses) -> PWM/1
  Constant/1 -> Divide/2
  Divide/1 -> "Compute time duration of switching states (Ta,Tb,To) "/2(m)
  "Determine the sector of U* based on alpha (rad). Also, determine if the sector number is odd"/2(Odd_S) -> Scope1/2, Display1/1, "Compute time duration of switching states (Ta,Tb,To) "/4(Odd_S)
  "Determine the sector of U* based on alpha (rad). Also, determine if the sector number is odd"/1(Sn) -> Generate pulse pattern/1(Sn), "Compute time duration of switching states (Ta,Tb,To) "/3(Sn), Scope1/1, Display/1
  Cartesian to Polar/1 -> Scope/1, Divide/1
  "Compute time duration of switching states (Ta,Tb,To) "/1(Ta_Tb_To) -> Scope2/1, Display2/1, Generate pulse pattern/2(TaTbTo)
  Ux/1 -> Cartesian to Polar/1
  Uy/1 -> Cartesian to Polar/2
  MATLAB Function/1(alpha_out) -> "Compute time duration of switching states (Ta,Tb,To) "/1(alpha), Scope/3, "Determine the sector of U* based on alpha (rad). Also, determine if the sector number is odd"/1(alpha)
  Cartesian to Polar/2 -> MATLAB Function/1(alpha), Scope/2

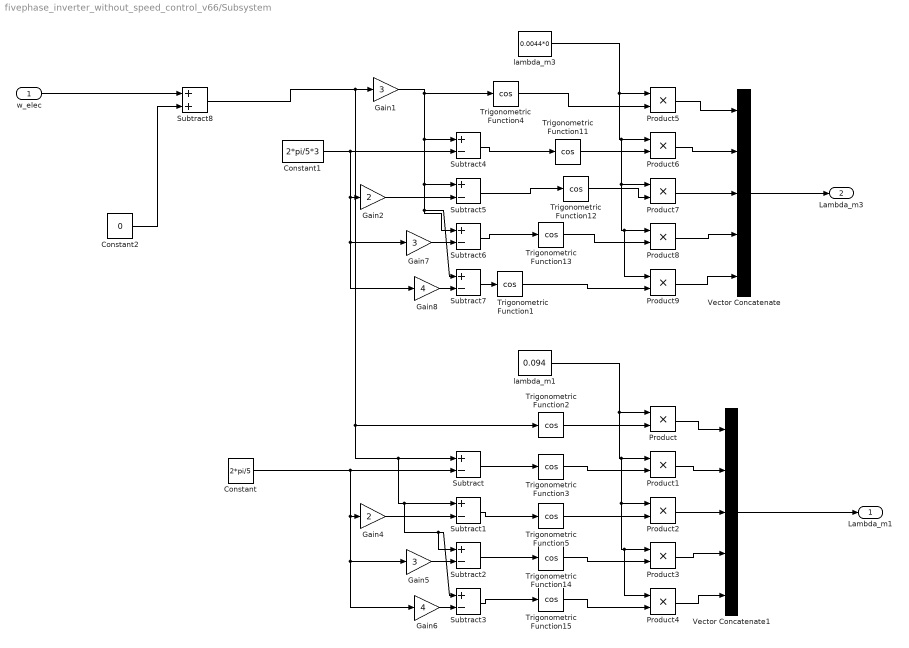
== system fivephase_inverter_without_speed_control_v66/Subsystem ==
  "w_elec " : Inport
  Constant : Constant  Value=2*pi/5
  Constant1 : Constant  Value=2*pi/5*3
  Constant2 : Constant  Value=0
  Gain1 : Gain  Gain=3
  Gain2 : Gain  Gain=2
  Gain4 : Gain  Gain=2
  Gain5 : Gain  Gain=3
  Gain6 : Gain  Gain=4
  Gain7 : Gain  Gain=3
  Gain8 : Gain  Gain=4
  Product{,1..9} (10 alike) : Product
  Subtract{,1..7} (8 alike) : Sum  Inputs=+-
  Subtract8 : Sum
  Trigonometric Function{1..5,11..15} (10 alike) : Trigonometry  Operator=cos
  Vector Concatenate : Concatenate  NumInputs=5
  Vector Concatenate1 : Concatenate  NumInputs=5
  "lambda_m1 " : Constant  Value=0.094
  lambda_m3 : Constant  Value=0.0044*0
  Lambda_m1 : Outport
  Lambda_m3 : Outport  Port=2
  wires:
  Gain4/1 -> Subtract1/2
  Gain6/1 -> Subtract3/2
  Gain5/1 -> Subtract2/2
  Subtract2/1 -> Trigonometric Function14/1
  Subtract3/1 -> Trigonometric Function15/1
  Subtract/1 -> Trigonometric Function3/1
  Subtract1/1 -> Trigonometric Function5/1
  Product/1 -> Vector Concatenate1/1
  Product1/1 -> Vector Concatenate1/2
  Product2/1 -> Vector Concatenate1/3
  Product3/1 -> Vector Concatenate1/4
  Product4/1 -> Vector Concatenate1/5
  "lambda_m1 "/1 -> Product4/1, Product3/1, Product2/1, Product1/1, Product/1
  Subtract4/1 -> Trigonometric Function11/1
  Product7/1 -> Vector Concatenate/3
  Gain2/1 -> Subtract5/2
  lambda_m3/1 -> Product9/1, Product8/1, Product7/1, Product6/1, Product5/1
  Gain7/1 -> Subtract6/2
  Gain8/1 -> Subtract7/2
  Subtract7/1 -> Trigonometric Function1/1
  Constant1/1 -> Gain8/1, Gain7/1, Gain2/1, Subtract4/2
  Product6/1 -> Vector Concatenate/2
  Product5/1 -> Vector Concatenate/1
  Trigonometric Function4/1 -> Product5/2
  Product8/1 -> Vector Concatenate/4
  Subtract5/1 -> Trigonometric Function12/1
  Trigonometric Function1/1 -> Product9/2
  Gain1/1 -> Trigonometric Function4/1, Subtract7/1, Subtract6/1, Subtract5/1, Subtract4/1
  Product9/1 -> Vector Concatenate/5
  Vector Concatenate1/1 -> Lambda_m1/1
  Vector Concatenate/1 -> Lambda_m3/1
  Constant/1 -> Gain6/1, Gain5/1, Gain4/1, Subtract/2
  Subtract8/1 -> Trigonometric Function2/1, Subtract3/1, Subtract2/1, Subtract1/1, Subtract/1, Gain1/1
  Constant2/1 -> Subtract8/2
  "w_elec "/1 -> Subtract8/1
  Trigonometric Function11/1 -> Product6/2
  Trigonometric Function12/1 -> Product7/2
  Subtract6/1 -> Trigonometric Function13/1
  Trigonometric Function13/1 -> Product8/2
  Trigonometric Function2/1 -> Product/2
  Trigonometric Function3/1 -> Product1/2
  Trigonometric Function5/1 -> Product2/2
  Trigonometric Function14/1 -> Product3/2
  Trigonometric Function15/1 -> Product4/2

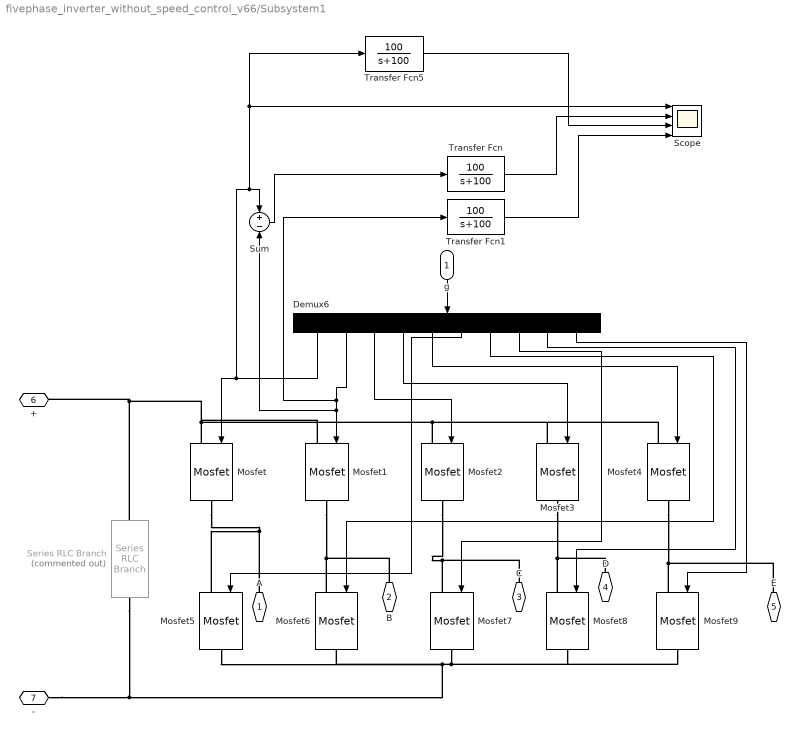
== system fivephase_inverter_without_speed_control_v66/Subsystem1 ==
  g : Inport
  Demux6 : Demux  Outputs=10
  Mosfet{,1..9} (10 alike) : powerlib/Power Electronics/Mosfet  Ron=0.1  Lon=0  Rd=0.01  Vfd=0  IC=0  Rs=1e5  Cs=inf  Measurements=off
      settings: SourceProductName=Simscape Electrical
  Scope : Scope  NumInputPorts=4
  Series RLC Branch : powerlib/Elements/Series RLC Branch  Commented=on  LConnTagsString=__new0  RConnTagsString=__new0  BranchType=C  Resistance=1  Inductance=1e-3  SetiL0=off  InitialCurrent=0  Capacitance=1e-6  Setx0=off  InitialVoltage=0  Measurements=None
      settings: SourceProductName=Simscape Electrical
  Sum : Sum  Inputs=+-
  Transfer Fcn : TransferFcn  Numerator=[100]  Denominator=[1 100]
  Transfer Fcn1 : TransferFcn  Numerator=[100]  Denominator=[1 100]
  Transfer Fcn5 : TransferFcn  Numerator=[100]  Denominator=[1 100]
  A : PMIOPort  Side=Right
  B : PMIOPort  Port=2  Side=Right
  C : PMIOPort  Port=3  Side=Right
  D : PMIOPort  Port=4  Side=Right
  E : PMIOPort  Port=5  Side=Right
  + : PMIOPort  Port=6  Side=Left
  - : PMIOPort  Port=7  Side=Left
  wires:
  g/1 -> Demux6/1
  Demux6/1 -> Mosfet/1, Transfer Fcn5/1, Scope/1, Sum/1
  Demux6/2 -> Transfer Fcn1/1, Mosfet1/1, Sum/2
  Demux6/3 -> Mosfet2/1
  Demux6/5 -> Mosfet4/1
  Demux6/6 -> Mosfet5/1
  Demux6/7 -> Mosfet6/1
  Demux6/8 -> Mosfet7/1
  Demux6/9 -> Mosfet8/1
  Demux6/10 -> Mosfet9/1
  Sum/1 -> Transfer Fcn/1
  Transfer Fcn/1 -> Scope/2
  Demux6/4 -> Mosfet3/1
  Transfer Fcn5/1 -> Scope/3
  Transfer Fcn1/1 -> Scope/4
  connections:
  E/RConn1 -- Mosfet9/LConn1 -- Mosfet4/RConn1
  D/RConn1 -- Mosfet8/LConn1 -- Mosfet3/RConn1
  C/RConn1 -- Mosfet2/RConn1 -- Mosfet7/LConn1
  B/RConn1 -- Mosfet6/LConn1 -- Mosfet1/RConn1
  A/RConn1 -- Mosfet5/LConn1 -- Mosfet/RConn1
  Mosfet2/LConn1 -- Mosfet4/LConn1 -- Mosfet3/LConn1 -- Mosfet/LConn1 -- Mosfet1/LConn1 -- +/RConn1 -- Series RLC Branch/LConn1
  -/RConn1 -- Series RLC Branch/RConn1 -- Mosfet5/RConn1 -- Mosfet6/RConn1 -- Mosfet7/RConn1 -- Mosfet8/RConn1 -- Mosfet9/RConn1

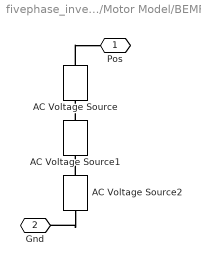
== system fivephase_inverter_without_speed_control_v66/Motor Model/BEMF5 ==
  AC Voltage Source : powerlib/Electrical Sources/AC Voltage Source  Amplitude=fund  Phase=phase  Frequency=freq  SampleTime=0  Measurements=None  BusType=swing  Pref=10e3  Qref=0  Qmin=-inf  Qmax=+inf
      settings: SourceProductName=Simscape Electrical
  AC Voltage Source1 : powerlib/Electrical Sources/AC Voltage Source  Amplitude=third  Phase=phase*3  Frequency=freq*3  SampleTime=0  Measurements=None  BusType=swing  Pref=10e3  Qref=0  Qmin=-inf  Qmax=+inf
      settings: SourceProductName=Simscape Electrical
  AC Voltage Source2 : powerlib/Electrical Sources/AC Voltage Source  Amplitude=fifth  Phase=phase*5  Frequency=freq*5  SampleTime=0  Measurements=None  BusType=swing  Pref=10e3  Qref=0  Qmin=-inf  Qmax=+inf
      settings: SourceProductName=Simscape Electrical
  Pos : PMIOPort  Side=Right
  Gnd : PMIOPort  Port=2  Side=Left
  connections:
  AC Voltage Source2/LConn1 -- Gnd/RConn1
  AC Voltage Source1/RConn1 -- AC Voltage Source/LConn1
  AC Voltage Source/RConn1 -- Pos/RConn1
  AC Voltage Source2/RConn1 -- AC Voltage Source1/LConn1

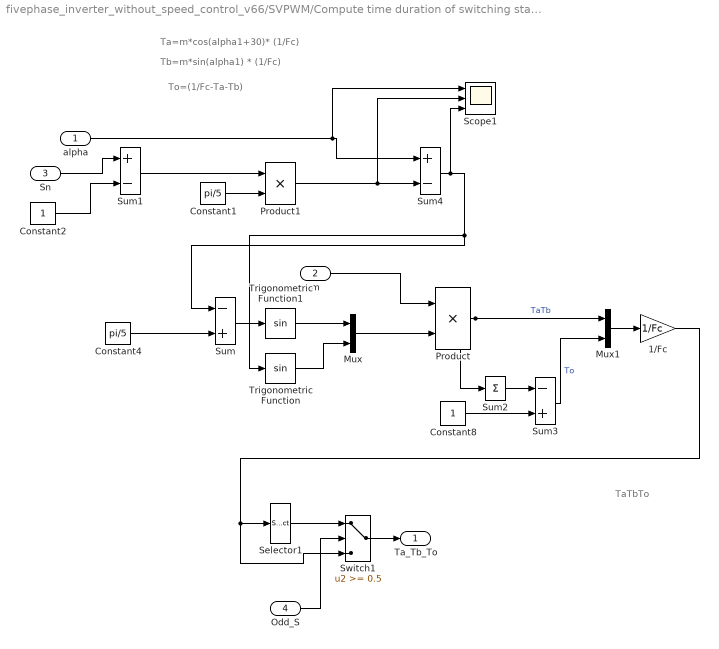
== system fivephase_inverter_without_speed_control_v66/SVPWM/Compute time duration of switching states (Ta,Tb,To)  ==
  note: TaTbTo
  note: To=(1/Fc-Ta-Tb)
  note: Tb=m*sin(alpha1) * (1/Fc)
  note: Ta=m*cos(alpha1+30)* (1/Fc)
  alpha : Inport
  m : Inport  Port=2
  Sn : Inport  Port=3
  Odd_S : Inport  Port=4
  1/Fc : Gain  Gain=1/Fc  SaturateOnIntegerOverflow=on  OutDataTypeStr=Inherit: Same as input  ParamDataTypeStr=Inherit: Same as input
  Constant1 : Constant  Value=pi/5
  Constant2 : Constant
  Constant4 : Constant  Value=pi/5
  Constant8 : Constant
  Mux : Mux  Inputs=2
  Mux1 : Mux  Inputs=2
  Product : Product  SaturateOnIntegerOverflow=on  OutDataTypeStr=Inherit: Same as first input
  Product1 : Product  SaturateOnIntegerOverflow=on  OutDataTypeStr=Inherit: Same as first input
  Scope1 : Scope  NumInputPorts=3
  Selector1 : Selector  InputPortWidth=3  IndexOptions=Index vector (dialog)  Indices=[2 1 3]  OutputSizes=1
  Sum : Sum  Inputs=-+  SaturateOnIntegerOverflow=on
  Sum1 : Sum  Inputs=+-  SaturateOnIntegerOverflow=on
  Sum2 : Sum  Inputs=1  SaturateOnIntegerOverflow=on
  Sum3 : Sum  Inputs=-+  SaturateOnIntegerOverflow=on
  Sum4 : Sum  Inputs=+-  SaturateOnIntegerOverflow=on
  Switch1 : Switch  Threshold=0.5  SaturateOnIntegerOverflow=on
  Trigonometric Function : Trigonometry
  Trigonometric Function1 : Trigonometry
  Ta_Tb_To : Outport
  wires:
  Switch1/1 -> Ta_Tb_To/1
  Mux1/1 -> 1/Fc/1
  Sum3/1 -> Mux1/2  "To"
  Product/1 -> Sum2/1, Mux1/1  "TaTb"
  Product1/1 -> Scope1/2, Sum4/2
  Constant1/1 -> Product1/2
  Constant8/1 -> Sum3/2
  Sum2/1 -> Sum3/1
  Sum/1 -> Trigonometric Function1/1
  m/1 -> Product/1
  Constant4/1 -> Sum/2
  Odd_S/1 -> Switch1/2
  Mux/1 -> Product/2
  alpha/1 -> Scope1/1, Sum4/1
  Sum4/1 -> Trigonometric Function/1, Sum/1, Scope1/3
  1/Fc/1 -> Switch1/3, Selector1/1
  Constant2/1 -> Sum1/2
  Sn/1 -> Sum1/1
  Sum1/1 -> Product1/1
  Trigonometric Function/1 -> Mux/2
  Trigonometric Function1/1 -> Mux/1
  Selector1/1 -> Switch1/1

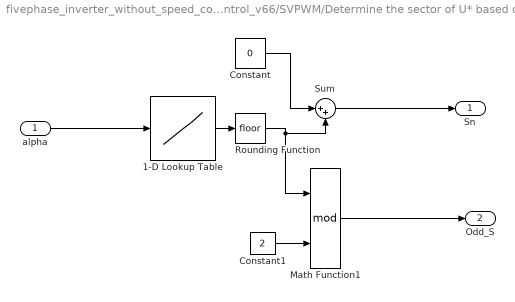
== system fivephase_inverter_without_speed_control_v66/SVPWM/Determine the sector of U* based on alpha (rad). Also, determine if the sector number is odd ==
  alpha : Inport
  1-D Lookup Table : Lookup_n-D  NumberOfTableDimensions=1  BreakpointsForDimension1=[0:pi/5:9*pi/5]  BeginIndexSearchUsingPreviousIndexResult=on  Table=[1:10]  InternalRulePriority=Speed  RndMeth=Simplest  InputSameDT=on
  Constant : Constant  Value=0
  Constant1 : Constant  Value=2
  Math Function1 : Math  Operator=mod  SaturateOnIntegerOverflow=on
  Rounding Function : Rounding
  Sum : Sum  Inputs=|++
  Sn : Outport
  Odd_S : Outport  Port=2
  wires:
  Math Function1/1 -> Odd_S/1
  Constant1/1 -> Math Function1/2
  Rounding Function/1 -> Sum/2, Math Function1/1
  1-D Lookup Table/1 -> Rounding Function/1
  Constant/1 -> Sum/1
  Sum/1 -> Sn/1
  alpha/1 -> 1-D Lookup Table/1

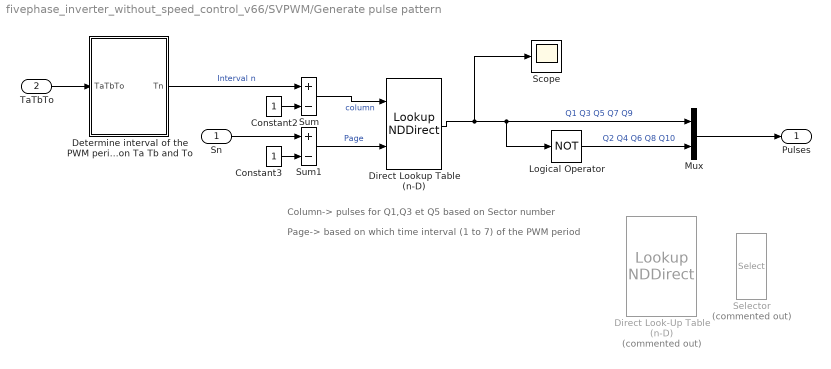
== system fivephase_inverter_without_speed_control_v66/SVPWM/Generate pulse pattern ==
  note: Column-> pulses for Q1,Q3 et Q5 based on Sector number
  note: Page-> based on which time interval (1 to 7) of the PWM period
  Sn : Inport
  TaTbTo : Inport  Port=2
  Constant2 : Constant  SampleTime=Ts
  Constant3 : Constant  SampleTime=Ts
  Determine interval of the PWM period based on Ta Tb and To : Subsystem
  Direct Look-Up Table (n-D) : LookupNDDirect  Commented=on  NumberOfTableDimensions=3  InputsSelectThisObjectFromTable=Vector  Table=pat1
  Direct Lookup Table (n-D) : LookupNDDirect  NumberOfTableDimensions=3  InputsSelectThisObjectFromTable=Vector  Table=pulse
  Logical Operator : Logic  Operator=NOT  AllPortsSameDT=off  OutDataTypeStr=float('double')
  Mux : Mux  Inputs=[5 5]
  Scope : Scope
  Selector : Selector  Commented=on  InputPortWidth=6  IndexOptions=Index vector (dialog)  Indices=[1 4 2 5 3 6]  OutputSizes=1
  Sum : Sum  Inputs=+-  SaturateOnIntegerOverflow=on
  Sum1 : Sum  Inputs=+-  SaturateOnIntegerOverflow=on
  Pulses : Outport
  wires:
  TaTbTo/1 -> Determine interval of the PWM period based on Ta Tb and To/1(TaTbTo)
  Constant2/1 -> Sum/2
  Constant3/1 -> Sum1/2
  Sn/1 -> Sum1/1
  Direct Lookup Table (n-D)/1 -> Scope/1, Logical Operator/1, Mux/1  "Q1 Q3 Q5 Q7 Q9"
  Logical Operator/1 -> Mux/2  "Q2 Q4 Q6 Q8 Q10"
  Mux/1 -> Pulses/1
  Determine interval of the PWM period based on Ta Tb and To/1(Tn) -> Sum/1  "Interval n"
  Sum1/1 -> Direct Lookup Table (n-D)/2  "Page"
  Sum/1 -> Direct Lookup Table (n-D)/1  "column"

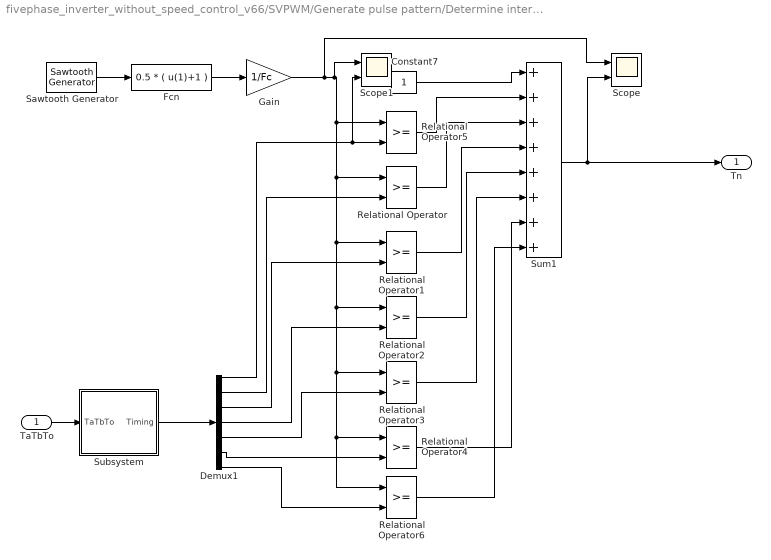
== system fivephase_inverter_without_speed_control_v66/SVPWM/Generate pulse pattern/Determine interval of the PWM period based on Ta Tb and To ==
  TaTbTo : Inport
  Constant7 : Constant  SampleTime=Ts
  Demux1 : Demux  Outputs=7
  Fcn : Fcn  Expr=0.5 * ( u(1)+1 )
  Gain : Gain  Gain=1/Fc
  Relational Operator{,1..6} (7 alike) : RelationalOperator  RndMeth=Nearest
  Sawtooth Generator : powerlib_meascontrol/Pulse & Signal Generators/Sawtooth Generator  Freq=Fc  Phase=0  Ts=Ts
      settings: SourceProductName=Simscape Electrical
  Scope : Scope  NumInputPorts=2
  Scope1 : Scope  NumInputPorts=2
  Subsystem : Subsystem
  Sum1 : Sum  Inputs=++++++++  SaturateOnIntegerOverflow=on
  Tn : Outport
  wires:
  Sawtooth Generator/1 -> Fcn/1
  TaTbTo/1 -> Subsystem/1(TaTbTo)
  Subsystem/1(Timing) -> Demux1/1
  Relational Operator4/1 -> Sum1/7
  Relational Operator3/1 -> Sum1/6
  Relational Operator2/1 -> Sum1/5
  Relational Operator1/1 -> Sum1/4
  Relational Operator/1 -> Sum1/3
  Relational Operator5/1 -> Sum1/2
  Constant7/1 -> Sum1/1
  Demux1/1 -> Scope1/2, Relational Operator5/2
  Demux1/2 -> Relational Operator/2
  Demux1/3 -> Relational Operator1/2
  Demux1/4 -> Relational Operator2/2
  Demux1/5 -> Relational Operator3/2
  Demux1/6 -> Relational Operator4/2
  Sum1/1 -> Tn/1, Scope/2
  Fcn/1 -> Gain/1
  Demux1/7 -> Relational Operator6/2
  Gain/1 -> Scope/1, Scope1/1, Relational Operator6/1, Relational Operator4/1, Relational Operator3/1, Relational Operator2/1, Relational Operator1/1, Relational Operator/1, Relational Operator5/1
  Relational Operator6/1 -> Sum1/8

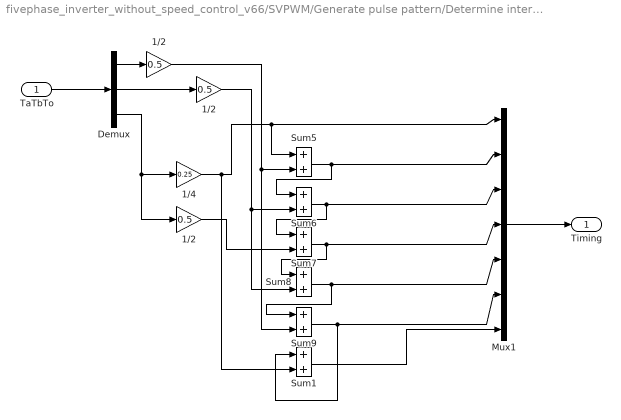
== system fivephase_inverter_without_speed_control_v66/SVPWM/Generate pulse pattern/Determine interval of the PWM period based on Ta Tb and To/Subsystem ==
  TaTbTo : Inport
  "  1/2" : Gain  Gain=0.5  SaturateOnIntegerOverflow=on  OutDataTypeStr=Inherit: Same as input  ParamDataTypeStr=Inherit: Same as input
  " 1/2" : Gain  Gain=0.5  SaturateOnIntegerOverflow=on  OutDataTypeStr=Inherit: Same as input  ParamDataTypeStr=Inherit: Same as input
  " 1/2 " : Gain  Gain=0.5  SaturateOnIntegerOverflow=on  OutDataTypeStr=Inherit: Same as input  ParamDataTypeStr=Inherit: Same as input
  1/4 : Gain  Gain=0.25  SaturateOnIntegerOverflow=on  OutDataTypeStr=Inherit: Same as input  ParamDataTypeStr=Inherit: Same as input
  Demux : Demux  Outputs=3
  Mux1 : Mux  Inputs=7
  Sum{1,5..9} (6 alike) : Sum  SaturateOnIntegerOverflow=on
  Timing : Outport
  wires:
  " 1/2 "/1 -> Sum9/2, Sum5/2
  Demux/3 -> " 1/2"/1, 1/4/1
  "  1/2"/1 -> Sum8/2, Sum6/2
  TaTbTo/1 -> Demux/1
  " 1/2"/1 -> Sum7/2
  1/4/1 -> Sum1/2, Sum5/1, Mux1/1
  Sum9/1 -> Sum1/1, Mux1/6
  Sum8/1 -> Sum9/1, Mux1/5
  Sum7/1 -> Sum8/1, Mux1/4
  Sum6/1 -> Sum7/1, Mux1/3
  Sum5/1 -> Sum6/1, Mux1/2
  Mux1/1 -> Timing/1
  Sum1/1 -> Mux1/7
  Demux/1 -> " 1/2 "/1
  Demux/2 -> "  1/2"/1

== matlab function fivephase_inverter_without_speed_control_v66/MATLAB Function1 ==
  data: Ia input; d1 output; Ib input; Ic input; Id input; Ie input; theta input; q1 output; d3 output; q3 output; zero output
function [d1,q1,d3,q3,zero] = abcde2dq(Ia,Ib,Ic,Id,Ie,theta)
% d1 = 0;
% q1 = 0;
% d3 = 0;
% q3 = 0;
% zero = 0;

I_5ph = [Ia;Ib;Ic;Id;Ie];

T = 2/5*...
    [cos(theta),cos(theta-2*pi/5),cos(theta-4*pi/5),cos(theta-6*pi/5),cos(theta-8*pi/5);
    -sin(theta),-sin(theta-2*pi/5),-sin(theta-4*pi/5),-sin(theta-6*pi/5),-sin(theta-8*pi/5);
    cos(3*theta),cos(3*theta-6*pi/5),cos(3*theta-2*pi/5),cos(3*theta-8*pi/5),cos(3*theta-4*pi/5);
    -sin(3*theta),-sin(3*theta-6*pi/5),-sin(3*theta-2*pi/5),-sin(3*theta-8*pi/5),-sin(3*theta-4*pi/5);
    1/sqrt(2), 1/sqrt(2),        1/sqrt(2),        1/sqrt(2),        1/sqrt(2)];

Iqd = T*I_5ph;
d1 = Iqd(1);
q1 = Iqd(2);
d3 = Iqd(3);
q3 = Iqd(4);
zero = Iqd(5);
end

== matlab function fivephase_inverter_without_speed_control_v66/MATLAB Function ==
  data: Ia input; d1 output; Ib input; Ic input; Id input; Ie input; theta input; q1 output; d3 output; q3 output; zero output
function [d1,q1,d3,q3,zero] = abcde2dq(Ia,Ib,Ic,Id,Ie,theta)
% d1 = 0;
% q1 = 0;
% d3 = 0;
% q3 = 0;
% zero = 0;

I_5ph = [Ia;Ib;Ic;Id;Ie];

T = 2/5*...
    [cos(theta),cos(theta-2*pi/5),cos(theta-4*pi/5),cos(theta-6*pi/5),cos(theta-8*pi/5);
    -sin(theta),-sin(theta-2*pi/5),-sin(theta-4*pi/5),-sin(theta-6*pi/5),-sin(theta-8*pi/5);
    cos(3*theta),cos(3*theta-6*pi/5),cos(3*theta-2*pi/5),cos(3*theta-8*pi/5),cos(3*theta-4*pi/5);
    -sin(3*theta),-sin(3*theta-6*pi/5),-sin(3*theta-2*pi/5),-sin(3*theta-8*pi/5),-sin(3*theta-4*pi/5);
    1/sqrt(2), 1/sqrt(2),        1/sqrt(2),        1/sqrt(2),        1/sqrt(2)];


Iqd = T*I_5ph;
d1 = Iqd(1);
q1 = Iqd(2);
d3 = Iqd(3);
q3 = Iqd(4);
zero = Iqd(5);
end

== matlab function fivephase_inverter_without_speed_control_v66/MATLAB Function2 ==
  data: Id1 input; a output; Iq1 input; Id3 input; Iq3 input; zero input; theta input; b output; c output; d output; e output
function [a,b,c,d,e] = dq2abcde(Id1,Iq1,Id3,Iq3,zero,theta)
I_dq= [Id1;Iq1;Id3;Iq3;zero];
T = 2/5*...
    [cos(theta),cos(theta-2*pi/5),cos(theta-4*pi/5),cos(theta-6*pi/5),cos(theta-8*pi/5);
    -sin(theta),-sin(theta-2*pi/5),-sin(theta-4*pi/5),-sin(theta-6*pi/5),-sin(theta-8*pi/5);
    cos(3*theta),cos(3*theta-6*pi/5),cos(3*theta-2*pi/5),cos(3*theta-8*pi/5),cos(3*theta-4*pi/5);
    -sin(3*theta),-sin(3*theta-6*pi/5),-sin(3*theta-2*pi/5),-sin(3*theta-8*pi/5),-sin(3*theta-4*pi/5);
    1/sqrt(2), 1/sqrt(2),        1/sqrt(2),        1/sqrt(2),        1/sqrt(2)];


Tinv = @(theta) T(theta)'*5/2;

Tinv = 5/2*T';

I_5ph = Tinv * I_dq;
a = I_5ph(1);
b = I_5ph(2);
c = I_5ph(3);
d = I_5ph(4);
e = I_5ph(5);

end

== matlab function fivephase_inverter_without_speed_control_v66/MATLAB Function3 ==
  data: Id1 input; a output; Iq1 input; Id3 input; Iq3 input; zero input; theta input; b output; c output; d output; e output
function [a,b,c,d,e] = dq2abcde(Id1,Iq1,Id3,Iq3,zero,theta)
I_dq= [Id1;Iq1;Id3;Iq3;zero];

T = 2/5*...
    [cos(theta),cos(theta-2*pi/5),cos(theta-4*pi/5),cos(theta-6*pi/5),cos(theta-8*pi/5);
    -sin(theta),-sin(theta-2*pi/5),-sin(theta-4*pi/5),-sin(theta-6*pi/5),-sin(theta-8*pi/5);
    cos(3*theta),cos(3*theta-6*pi/5),cos(3*theta-2*pi/5),cos(3*theta-8*pi/5),cos(3*theta-4*pi/5);
    -sin(3*theta),-sin(3*theta-6*pi/5),-sin(3*theta-2*pi/5),-sin(3*theta-8*pi/5),-sin(3*theta-4*pi/5);
    1/sqrt(2), 1/sqrt(2),        1/sqrt(2),        1/sqrt(2),        1/sqrt(2)];


Tinv = @(theta) T(theta)'*5/2;

Tinv = 5/2*T';

I_5ph = Tinv * I_dq;
a = I_5ph(1);
b = I_5ph(2);
c = I_5ph(3);
d = I_5ph(4);
e = I_5ph(5);

end

== matlab function fivephase_inverter_without_speed_control_v66/SVPWM/MATLAB Function ==
  data: alpha input; alpha_out output
function alpha_out = angle_correction(alpha)

alpha_out = alpha;

if alpha < 0
    alpha_out = alpha +2*pi;
end
if alpha >= 0
    alpha_out = alpha;
    
end
end
